simulink model "esettest"  (Simulink 6.5)
settings: Solver=FixedStepDiscrete  StartTime=0.0  StopTime=inf  FixedStep=0.04  RelTol=1e-3
libraries: StandardLib x10, simulink x2, WindLib x2
settings Model: Creator=204050978  LastModifiedBy=204050978

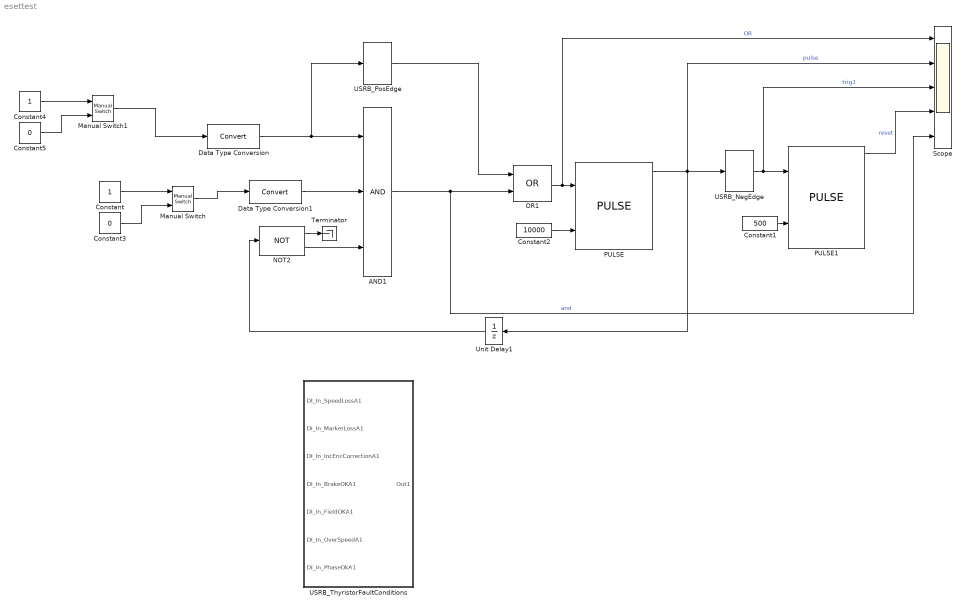
== system esettest ==
  AND1 : StandardLib/Logical operations/AND  RepeatCnt=2  SampleTime=-1  ExecutionOrder=0
  Constant : Constant  Value=1  OutDataType=sfix(16)  ConRadixGroup=Use specified scaling  OutScaling=2^0  SampleTime=inf  FramePeriod=inf
  Constant1 : Constant  Value=500  OutDataTypeMode=uint32  OutDataType=sfix(16)  ConRadixGroup=Use specified scaling  OutScaling=2^0  SampleTime=inf  FramePeriod=inf
  Constant2 : Constant  Value=10000  OutDataTypeMode=uint32  OutDataType=sfix(16)  ConRadixGroup=Use specified scaling  OutScaling=2^0  SampleTime=inf  FramePeriod=inf
  Constant3 : Constant  Value=0  OutDataType=sfix(16)  ConRadixGroup=Use specified scaling  OutScaling=2^0  SampleTime=inf  FramePeriod=inf
  Constant4 : Constant  Value=1  OutDataType=sfix(16)  ConRadixGroup=Use specified scaling  OutScaling=2^0  SampleTime=inf  FramePeriod=inf
  Constant5 : Constant  Value=0  OutDataType=sfix(16)  ConRadixGroup=Use specified scaling  OutScaling=2^0  SampleTime=inf  FramePeriod=inf
  Data Type Conversion : DataTypeConversion  OutDataTypeMode=boolean
  Data Type Conversion1 : DataTypeConversion  OutDataTypeMode=boolean
  Manual Switch : simulink/Signal Routing/Manual Switch  SystemSampleTime=-1  sw=1  action=0
  Manual Switch1 : simulink/Signal Routing/Manual Switch  SystemSampleTime=-1  sw=1  action=0
  NOT2 : StandardLib/Logical operations/NOT  SampleTime=-1  ExecutionOrder=0
  OR1 : StandardLib/Logical operations/OR  RepeatCnt=1  SampleTime=-1  ExecutionOrder=0
  PULSE : StandardLib/Sequencing/PULSE  SampleTime=-1  ExecutionOrder=0
  PULSE1 : StandardLib/Sequencing/PULSE  SampleTime=-1  ExecutionOrder=0
  Scope : Scope  NumInputPorts=5
      settings: TimeRange=10000  YMin=-5~-5~-5~-5~-5  YMax=5~5~5~5~5
  Terminator : Terminator
  USRB_NegEdge : WindLib/USRB_NegEdge  SystemSampleTime=-1
  USRB_PosEdge : WindLib/USRB_PosEdge  SystemSampleTime=-1
  USRB_ThyristorFaultConditions : Subsystem  TreatAsAtomicUnit=on
  Unit Delay1 : UnitDelay  Orientation=left  SampleTime=-1
  wires:
  Data Type Conversion/1 -> AND1/1, USRB_PosEdge/1
  PULSE/1 -> Unit Delay1/1, USRB_NegEdge/1, Scope/2  "pulse"
  Unit Delay1/1 -> NOT2/1
  Constant2/1 -> PULSE/2
  Constant1/1 -> PULSE1/2
  NOT2/2 -> AND1/3
  USRB_NegEdge/1 -> PULSE1/1, Scope/3  "trig1"
  NOT2/1 -> Terminator/1
  OR1/1 -> PULSE/1, Scope/1  "OR"
  AND1/1 -> OR1/2, Scope/5  "and"
  USRB_PosEdge/1 -> OR1/1
  PULSE1/1 -> Scope/4  "reset"
  Constant/1 -> Manual Switch/1
  Data Type Conversion1/1 -> AND1/2
  Manual Switch/1 -> Data Type Conversion1/1
  Constant3/1 -> Manual Switch/2
  Constant4/1 -> Manual Switch1/1
  Constant5/1 -> Manual Switch1/2
  Manual Switch1/1 -> Data Type Conversion/1

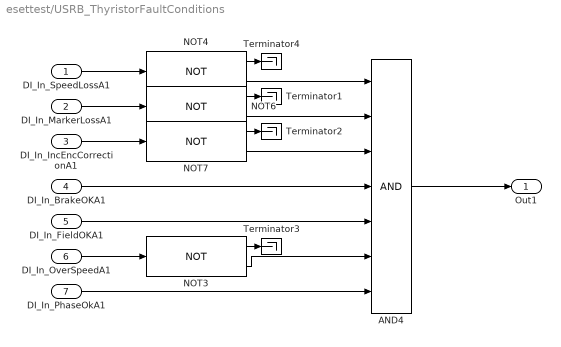
== system esettest/USRB_ThyristorFaultConditions ==
  DI_In_SpeedLossA1 : Inport  DataType=boolean
  DI_In_MarkerLossA1 : Inport  Port=2  DataType=boolean
  DI_In_IncEncCorrectionA1 : Inport  Port=3  DataType=boolean
  DI_In_BrakeOKA1 : Inport  Port=4  DataType=boolean
  DI_In_FieldOKA1 : Inport  Port=5  DataType=boolean
  DI_In_OverSpeedA1 : Inport  Port=6  DataType=boolean
  DI_In_PhaseOkA1 : Inport  Port=7  DataType=boolean
  AND4 : StandardLib/Logical operations/AND  RepeatCnt=6  SampleTime=-1  ExecutionOrder=0
  NOT{3..4,6..7} (4 alike) : StandardLib/Logical operations/NOT  SampleTime=-1  ExecutionOrder=0
  Terminator{1..4} (4 alike) : Terminator
  Out1 : Outport  DataType=boolean
  wires:
  AND4/1 -> Out1/1
  NOT3/1 -> Terminator3/1
  NOT3/2 -> AND4/6
  DI_In_OverSpeedA1/1 -> NOT3/1
  DI_In_PhaseOkA1/1 -> AND4/7
  DI_In_FieldOKA1/1 -> AND4/5
  DI_In_BrakeOKA1/1 -> AND4/4
  NOT7/1 -> Terminator2/1
  NOT6/1 -> Terminator1/1
  NOT4/1 -> Terminator4/1
  NOT7/2 -> AND4/3
  NOT6/2 -> AND4/2
  NOT4/2 -> AND4/1
  DI_In_IncEncCorrectionA1/1 -> NOT7/1
  DI_In_MarkerLossA1/1 -> NOT6/1
  DI_In_SpeedLossA1/1 -> NOT4/1
